simulink model "ECM_EKF_WLTP"  (R2021b)
settings: Solver=FixedStepDiscrete  StartTime=0.0  StopTime=10000  FixedStep=Ts_data  RelTol=1e-3
PreLoadFcn:
  | bdclose all
  | open_system('mdl/ECM_EKF_WLTP')
  | get_param(bdroot,'DataDictionary')
undefined symbols (not defined in the file or in its folder): C1_lut, C2_lut, crate_bp, DiscIntNeverNeededParam, R0_lut, R1_lut, R2_lut, raptor_get_param_eval, raptor_xcp_function, SoC0_guess, soc_bp, Ts_data
libraries: arc_dd_lib x12, Raptor_lib x8, arc_specialized_lib x4, simulink x2, arc_logic_lib x2, arc_fault_lib x2
(part 2 of 2)

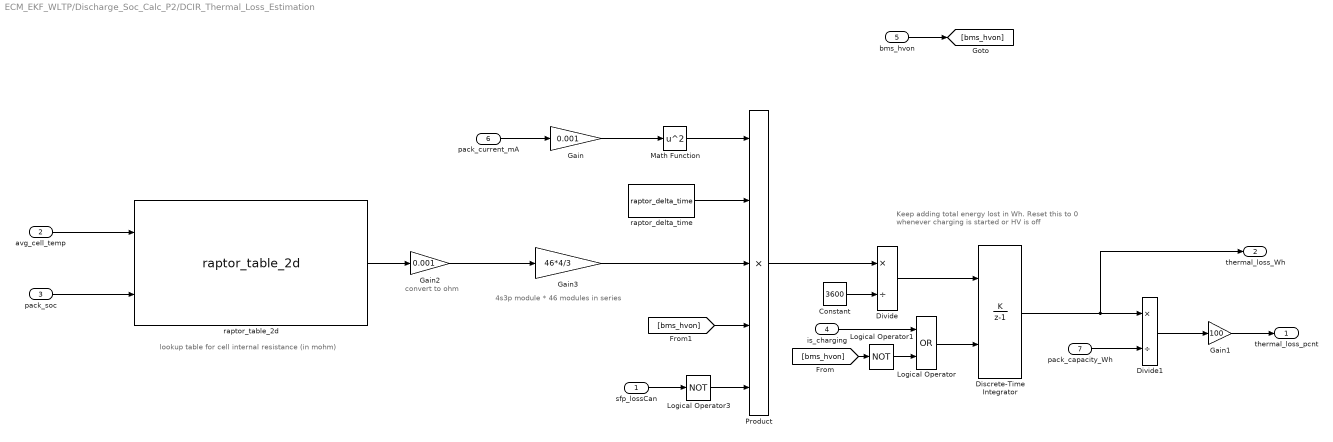
== system ECM_EKF_WLTP/Discharge_Soc_Calc_P2/DCIR_Thermal_Loss_Estimation ==
  note: 4s3p module * 46 modules in series
  note: convert to ohm
  note: lookup table for cell internal resistance (in mohm)
  note: Keep adding total energy lost in Wh. Reset this to 0 whenever charging is started or HV is off
  sfp_lossCan : Inport
  avg_cell_temp : Inport  Port=2
  pack_soc : Inport  Port=3
  is_charging : Inport  Port=4
  bms_hvon : Inport  Port=5
  pack_current_mA : Inport  Port=6
  pack_capacity_Wh : Inport  Port=7
  Constant : Constant  Value=3600
  Discrete-Time Integrator : DiscreteIntegrator  IntegratorMethod=Accumulation: Forward Euler  ExternalReset=level  SampleTime=-1  OutDataTypeStr=single  LimitOutput=on  UpperSaturationLimit=120000  LowerSaturationLimit=0  ICPrevOutput=DiscIntNeverNeededParam  ICPrevScaledInput=DiscIntNeverNeededParam
      settings: AttributesFormatString=|
      | %<UpperSaturationLimit>
      | %<LowerSaturationLimit>
  Divide : Product  Inputs=*/
  Divide1 : Product  Inputs=*/
  Gain : Gain  Gain=0.001
  Gain1 : Gain  Gain=100
  Gain2 : Gain  Gain=0.001
  Gain3 : Gain  Gain=46*4/3
  Logical Operator : Logic  Operator=OR  AllPortsSameDT=off  OutDataTypeStr=boolean
  Logical Operator1 : Logic  Operator=NOT  AllPortsSameDT=off  OutDataTypeStr=boolean
  Logical Operator3 : Logic  Operator=NOT  AllPortsSameDT=off  OutDataTypeStr=boolean
  Math Function : Math  Operator=square  SaturateOnIntegerOverflow=on
  Product : Product  Inputs=5
  raptor_delta_time : Raptor_lib/Triggers/raptor_delta_time  unit=seconds
      settings: SourceProductName=Raptor
  raptor_table_2d : Raptor_lib/Table Lookup/raptor_table_2d  dataName='dcir_p2'  initValue=|  dataType=double  storage=Calibration  initValueX=[5 10 15 20 25 30 35 40 45 50 55 60 65 70 75 80 85 90 95 100]  initValueY=[0 10 25 45]  dataTypeXY=double  storageXY=Calibration  calVisible=on  showTable=off  calGain=1.0  calOffset=0.0  calMax=Inf  calMin=-Inf  calFormat='-1'  calUnit=''  calHelp=''  showBreakpointX=off  dataNameX=[]  calGainX=1.0  calOffsetX=0.0  calMaxX=Inf  calMinX=-Inf  calFormatX='-1'  calUnitX=''  calHelpX=''  showBreakpointY=off  dataNameY=[]  calGainY=1.0  calOffsetY=0.0  calMaxY=Inf  calMinY=-Inf  calFormatY='-1'  calUnitY=''  calHelpY=''  calAccess=1  calFunction=raptor_xcp_function(gcb)  measureEnable=off  mName=[raptor_get_param_eval(gcb,'dataName'), '_Output']
      | [5.77000000000000	5.16400000000000	4.79100000000000	4.55700000000000	4.41700000000000	3.92700000000000	3.85800000000000	3.82300000000000	3.47000000000000	3.46700000000000	3.47200000000000	3.47900000000000	3.48400000000000	3.48600000000000	3.49400000000000	3.51100000000000	3.54500000000000	3.60100000000000	3.73100000000000	4.16700000000000;
      | 2.54900000000000	2.36200000000000	2.27500000000000	2.50700000000000	2.44900000000000	2.31500000000000	2.25000000000000	2.18000000000000	2.18500000000000	2.20700000000000	2.23300000000000	2.24600000000000	2.24200000000000	2.24000000000000	2.24800000000000	2.25000000000000	2.26100000000000	2.28500000000000	2.35800000000000	2.64100000000000;
      | 1.86600000000000	1.67500000000000	1.55200000000000	1.48700000000000	1.42900000000000	1.39400000000000	1.37700000000000	1.35600000000000	1.36400000000000	1.40000000000000	1.44500000000000	1.46200000000000	1.47000000000000	1.46800000000000	1.46100000000000	1.46800000000000	1.47100000000000	1.46800000000000	1.49800000000000	1.68000000000000;
      | 1.27500000000000	1.07800000000000	0.994000000000000	0.934000000000000	0.911000000000000	0.891000000000000	0.880000000000000	0.879000000000000	0.870000000000000	0.877000000000000	0.940000000000000	0.967000000000000	0.967000000000000	0.955000000000000	0.959000000000000	0.958000000000000	0.942000000000000	0.921000000000000	0.920000000000000	1.05600000000000]
      settings: SourceProductName=Raptor
  thermal_loss_pcnt : Outport
  thermal_loss_Wh : Outport  Port=2
  wires:
  pack_current_mA/1 -> Gain/1
  Math Function/1 -> Product/1
  raptor_delta_time/1 -> Product/2
  avg_cell_temp/1 -> raptor_table_2d/1
  pack_soc/1 -> raptor_table_2d/2
  raptor_table_2d/1 -> Gain2/1
  Gain/1 -> Math Function/1
  Product/1 -> Divide/1
  Constant/1 -> Divide/2
  Divide/1 -> Discrete-Time Integrator/1
  Logical Operator/1 -> Discrete-Time Integrator/2
  is_charging/1 -> Logical Operator/1
  Logical Operator1/1 -> Logical Operator/2
  bms_hvon/1 -> [bms_hvon]
  Discrete-Time Integrator/1 -> thermal_loss_Wh/1, Divide1/1
  pack_capacity_Wh/1 -> Divide1/2
  Divide1/1 -> Gain1/1
  Gain1/1 -> thermal_loss_pcnt/1
  [bms_hvon] -> Logical Operator1/1
  [bms_hvon] -> Product/4
  Logical Operator3/1 -> Product/5
  sfp_lossCan/1 -> Logical Operator3/1
  Gain2/1 -> Gain3/1
  Gain3/1 -> Product/3

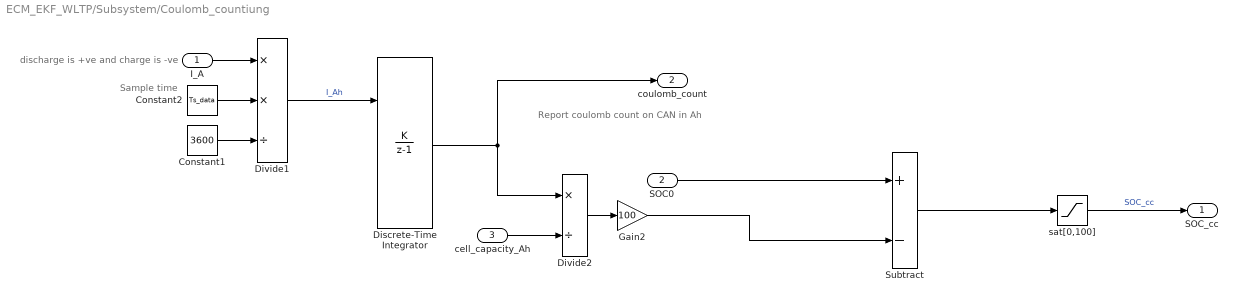
== system ECM_EKF_WLTP/Subsystem/Coulomb_countiung ==
  note: discharge is +ve and charge is -ve
  note: Report coulomb count on CAN in Ah
  note: Sample time
  I_A : Inport
  SOC0 : Inport  Port=2
  cell_capacity_Ah : Inport  Port=3
  Constant1 : Constant  Value=3600
  Constant2 : Constant  Value=Ts_data
  Discrete-Time Integrator : DiscreteIntegrator  IntegratorMethod=Accumulation: Forward Euler  ExternalReset=level  SampleTime=-1  LimitOutput=on  UpperSaturationLimit=175000  LowerSaturationLimit=-175000  ICPrevOutput=DiscIntNeverNeededParam  ICPrevScaledInput=DiscIntNeverNeededParam
      settings: AttributesFormatString=|
      | %<UpperSaturationLimit>
      | %<LowerSaturationLimit>
  Divide1 : Product  Inputs=**/
  Divide2 : Product  Inputs=*/
  Gain2 : Gain  Gain=100
  Subtract : Sum  Inputs=+-
  sat[0,100] : Saturate  UpperLimit=100  LowerLimit=0
  SOC_cc : Outport
  coulomb_count : Outport  Port=2
  wires:
  Divide1/1 -> Discrete-Time Integrator/1  "I_Ah"
  sat[0,100]/1 -> SOC_cc/1  "SOC_cc"
  Discrete-Time Integrator/1 -> coulomb_count/1, Divide2/1
  cell_capacity_Ah/1 -> Divide2/2
  Constant2/1 -> Divide1/2
  I_A/1 -> Divide1/1
  Divide2/1 -> Gain2/1
  Gain2/1 -> Subtract/2
  Subtract/1 -> sat[0,100]/1
  Constant1/1 -> Divide1/3
  SOC0/1 -> Subtract/1

== matlab function ECM_EKF_WLTP/Subsystem/MATLAB Function2 ==
  data: R2 input; Vrc1_next output; C2 input; Ts input; I input; Vrc2_prev input
function Vrc1_next = Vrc2_ZOH(R2, C2, Ts, I, Vrc2_prev)
% Exact ZOH update for fast RC branch
% Guards
R2 = min(max(R2, 1e-6), 10);
C2 = min(max(C2, 1e-6), 1e6);

tau1 = R2 * C2;
a    = exp( - Ts / tau1 );
b    = (1 - a) * R2;

Vrc1_next = a * Vrc2_prev + b * I;
end

== matlab function ECM_EKF_WLTP/Subsystem/MATLAB Function3 ==
  data: R input; V_next output; C input; Ts input; I_prev input; I_cur input; V_prev input; dIdt_thr input; force_mode input; mode_used output; a output

function [V_next, mode_used, a] = Vrc_FOHZOH(R, C, Ts, I_prev, I_cur, V_prev, dIdt_thr, force_mode)
% Hybrid FOH/ZOH update for a single RC branch, without charge-preservation.
% ZOH is exact for staircase inputs; FOH is exact for piecewise-linear ramps.

% ---------- Guards ----------
R  = min(max(R,  1e-6), 10);      % ohm
C  = min(max(C,  1e-6), 1e8);     % F (slow branch can be large)
Ts = max(Ts, 1e-6);               % s
tau = R * C;
a   = exp(-Ts / tau);             % exact decay factor

% ZOH (exact for holds): V[k] = a*V[k-1] + (1-a)*R*I[k-1]
Vzoh = a * V_prev + (1 - a) * R * I_prev;

% FOH (exact for ramps within the sample):
% Coefficients satisfy B_prev + B_cur = R*(1 - a)
B_prev = R - R * (tau/Ts) * (1 - a);
B_cur  = R * (tau/Ts) * (1 - a) - R * a;
Vfoh   = a * V_prev + B_prev * I_prev + B_cur * I_cur;

% ---------- Mode selection with hysteresis ----------
persistent last_mode
if isempty(last_mode), last_mode = 0; end             % start in ZOH
if force_mode == 0
    mode = 0;                                         % force ZOH
elseif force_mode == 1
    mode = 1;                                         % force FOH
else
    dIdt = (I_cur - I_prev) / Ts;
    if last_mode == 0 && abs(dIdt) > dIdt_thr
        mode = 1;                                     % ZOH -> FOH on strong ramp
    elseif last_mode == 1 && abs(dIdt) < 0.7 * dIdt_thr
        mode = 0;                                     % FOH -> ZOH when ramp weakens
    else
        mode = last_mode;                             % hold mode (avoid chatter)
    end
end

% ---------- Output ----------
V_next    = (mode==1) * Vfoh + (mode==0) * Vzoh;
mode_used = mode;
last_mode = mode;

% Optional clamp for sanity
V_next = min(max(V_next, -1e3), 1e3);
end
